simulink model "TetheredHelicopterControlAlgorithm"  (R2019a)
settings: Solver=ode5  StartTime=0.0  StopTime=50  FixedStep=0.01  RelTol=1e-3  AbsTol=1e-6
values from neighbouring files (symbols this model uses):
  Al = A    [Luenberg_matrix_calc.m]
  Bl = B    [Luenberg_matrix_calc.m]
  Cl = [1 0 0; 0 0 1]    [Luenberg_matrix_calc.m]
  fGain = KK(1)    [lqr_pitch.m]
  fi_0 = -0.63    [exp_pitch.m]    (also in linearization.m)
  L = transpose(place(transpose(Al),transpose(Cl),[-100.01,-100.02,-100.03]))    [Luenberg_matrix_calc.m]
  nGain = KK(3)    [lqr_pitch.m]
  pn1 = 1181    [lqr_eq_points.m]
  pn2 = -1053    [lqr_eq_points.m]
  pn3 = 990.5    [lqr_eq_points.m]
  pn4 = 1860    [lqr_eq_points.m]
  pu1 = 0.1721    [lqr_eq_points.m]
  pu2 = -0.1742    [lqr_eq_points.m]
  pu3 = 0.3003    [lqr_eq_points.m]
  pu4 = 0.364    [lqr_eq_points.m]
  wGain = KK(2)    [lqr_pitch.m]
undefined symbols (not defined in the file or in its folder): RTDAC4PCIBaseAddress
libraries: simulink x1, powerlib_meascontrol x1
settings Model: SimulationMode=external  ExtModeTrigDuration=12000  ExtModeTrigLevel=0.400000  Creator=jims  LastModifiedBy=User
settings SolverCC: AutoScaleAbsTol=off
settings DataIOCC: ExternalInput=[]  InitialState=[]  MaxDataPoints=5000  SaveFormat=Array  SignalLoggingSaveFormat=ModelDataLogs  SaveOutput=off  SaveTime=off  ReturnWorkspaceOutputs=off  SignalLoggingName=sigsOut
settings OptimizationCC: BooleanDataType=off  ExpressionDepthLimit=2147483647  InitFltsAndDblsToZero=on  LifeSpan=inf
settings DebuggingCC: SaveWithParameterizedLinksMsg=none  UnderspecifiedInitializationDetection=Classic  MergeDetectMultiDrivingBlocksExec=none  SignalResolutionControl=TryResolveAllWithWarning  MultiTaskDSMMsg=warning  MultiTaskCondExecSysMsg=none  IntegerOverflowMsg=none  FcnCallInpInsideContextMsg=warning  StateNameClashWarn=warning  SFUnexpectedBacktrackingDiag=warning  SFNoUnconditionalDefaultTransitionDiag=warning  SFExecutionAtInitializationDiag=none  IntegerSaturationMsg=none  ArithmeticOperatorsInVariantConditions=warning
settings HardwareCC: ProdBitPerLong=64  ProdLargestAtomicFloat=None  ProdHWDeviceType=Intel->x86-64  TargetBitPerLong=64  TargetBitPerPointer=64  TargetIntDivRoundTo=Zero  TargetEndianess=LittleEndian  TargetWordSize=64  TargetHWDeviceType=Intel->x86-64
settings ModelReferenceCC: PropagateSignalLabelsOutOfModel=off
settings SFSimCC: SimUseLocalCustomCode=off
settings RTWCC: SystemTargetFile=rtwin.tlc  TemplateMakefile=rtwin.tmf  Description=Real-Time Windows Target  RTWUseLocalCustomCode=off
settings CodeAppCC: StateflowObjectComments=on
settings TargetCC: TargetFcnLib=ansi_tfl_tmw.mat  TargetPreCompLibLocation=C:\Program Files\MATLAB\R2015aSP1\toolbox\sldrt\lib\win64  ModelReferenceCompliant=off  CompOptLevelCompliant=off  PreserveStateflowLocalDataDimensions=off
settings ConfigComp: CovMetricSettings=dw  CovHtmlReporting=on  CovSaveCumulativeToWorkspaceVar=on  CovSaveSingleToWorkspaceVar=on  CovExternalEMLEnable=off  CovSFcnEnable=off

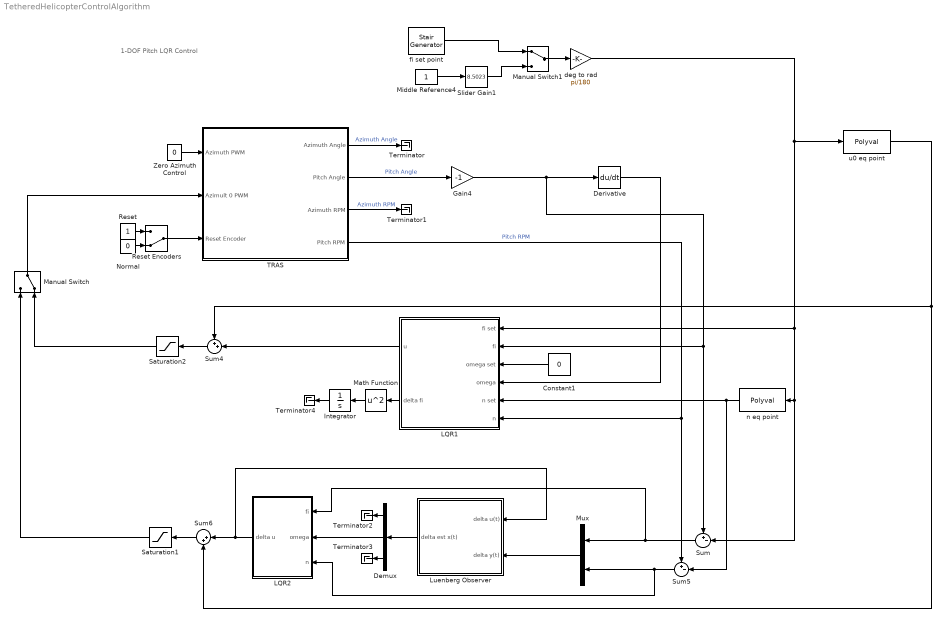
== system TetheredHelicopterControlAlgorithm ==
  note: 1-DOF Pitch LQR Control
  Constant1 : Constant  Value=0
  Demux : Demux  Outputs=3
  Derivative : Derivative
  Gain4 : Gain  Gain=-1
  Integrator : Integrator
  LQR1 : Subsystem
  "LQR2 " : Subsystem
  Luenberg Observer : Subsystem
  Manual Switch : ManualSwitch  CurrentSetting=0
  Manual Switch1 : ManualSwitch
  Math Function : Math  Operator=square  SaturateOnIntegerOverflow=on
  Middle Reference4 : Constant
  Mux : Mux  Inputs=2
  Normal : Constant  Value=0
  Reset : Constant
  Reset Encoders : ManualSwitch  CurrentSetting=0
  Saturation1 : Saturate  UpperLimit=1  LowerLimit=-1
  Saturation2 : Saturate  UpperLimit=1  LowerLimit=-1
  Slider Gain1 : simulink/Math Operations/Slider Gain  gain=8.5023  low=-45  high=45
  Sum : Sum  Inputs=+-|
  Sum4 : Sum  Inputs=++|  SaturateOnIntegerOverflow=on  InputSameDT=on  OutDataTypeStr=Inherit: Same as first input
  Sum5 : Sum  Inputs=+-|
  Sum6 : Sum  Inputs=|++  SaturateOnIntegerOverflow=on  InputSameDT=on  OutDataTypeStr=Inherit: Same as first input
  TRAS : Subsystem  mask{BaseAddress=RTDAC4PCIBaseAddress, T0=0.01}
      mask prompts: BaseAddress "Base Address:"; T0 "Sampling Period:"
      mask Display: image(imread('TRAS.JPG'))
  Terminator{,1..4} (5 alike) : Terminator
  Zero Azimuth Control : Constant  Value=0
  deg to rad : Gain  Gain=pi/180
  fi set point : powerlib_meascontrol/Pulse & Signal Generators/Stair Generator  t=[0 10 20 28 34 42]  e=[0 10 -20 20 -10 30]  Ts=0
      settings: SourceProductName=Simscape Electrical
  n eq point : Polyval  Coefs=[pn1 pn2 pn3 pn4]
  u0 eq point : Polyval  Coefs=[pu1 pu2 pu3 pu4]
  wires:
  TRAS/1(Azimuth Angle) -> Terminator/1  "Azimuth Angle"
  TRAS/2(Pitch Angle) -> Gain4/1  "Pitch Angle"
  TRAS/3(Azimuth RPM) -> Terminator1/1  "Azimuth RPM"
  Normal/1 -> Reset Encoders/2
  Reset/1 -> Reset Encoders/1
  Reset Encoders/1 -> TRAS/3(Reset Encoder)
  Zero Azimuth Control/1 -> TRAS/1(Azimuth PWM)
  TRAS/4(Pitch RPM) -> Sum5/1, LQR1/6(n)  "Pitch RPM"
  Gain4/1 -> Derivative/1, Sum/1, LQR1/2(fi)
  Constant1/1 -> LQR1/3(omega set)
  n eq point/1 -> LQR1/5(n set), Sum5/2
  Sum4/1 -> Saturation2/1
  Manual Switch1/1 -> deg to rad/1
  LQR1/1(u) -> Sum4/2
  Derivative/1 -> LQR1/4(omega)
  LQR1/2(delta fi) -> Math Function/1
  Math Function/1 -> Integrator/1
  Integrator/1 -> Terminator4/1
  u0 eq point/1 -> Sum4/1, Sum6/2
  Sum5/1 -> "LQR2 "/3(n), Mux/2
  Mux/1 -> Luenberg Observer/2(delta y(t))
  Luenberg Observer/1(delta est x(t)) -> Demux/1
  Sum6/1 -> Saturation1/1
  Saturation1/1 -> Manual Switch/1
  "LQR2 "/1("delta u ") -> Luenberg Observer/1(delta u(t)), Sum6/1
  Manual Switch/1 -> TRAS/2(Azimult 0 PWM)
  Saturation2/1 -> Manual Switch/2
  Middle Reference4/1 -> Slider Gain1/1
  Slider Gain1/1 -> Manual Switch1/2
  fi set point/1 -> Manual Switch1/1
  deg to rad/1 -> Sum/2, n eq point/1, LQR1/1(fi set), u0 eq point/1
  Sum/1 -> Mux/1, "LQR2 "/1(fi)
  Demux/2 -> "LQR2 "/2(omega)
  Demux/1 -> Terminator2/1
  Demux/3 -> Terminator3/1

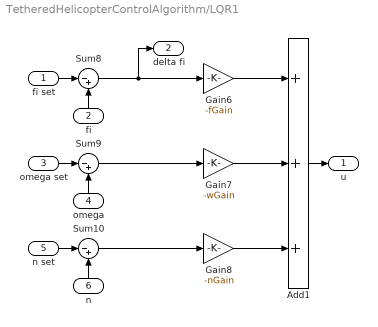
== system TetheredHelicopterControlAlgorithm/LQR1 ==
  fi set : Inport
  fi : Inport  Port=2
  omega set : Inport  Port=3
  omega : Inport  Port=4
  n set : Inport  Port=5
  n : Inport  Port=6
  Add1 : Sum  Inputs=+++
  Gain6 : Gain  Gain=-fGain
  Gain7 : Gain  Gain=-wGain
  Gain8 : Gain  Gain=-nGain
  Sum10 : Sum  Inputs=|-+
  Sum8 : Sum  Inputs=|-+
  Sum9 : Sum  Inputs=|-+
  u : Outport
  delta fi : Outport  Port=2
  wires:
  Gain7/1 -> Add1/2
  Sum8/1 -> delta fi/1, Gain6/1
  Sum9/1 -> Gain7/1
  Gain6/1 -> Add1/1
  Sum10/1 -> Gain8/1
  Gain8/1 -> Add1/3
  fi/1 -> Sum8/2
  n/1 -> Sum10/2
  n set/1 -> Sum10/1
  omega set/1 -> Sum9/1
  omega/1 -> Sum9/2
  Add1/1 -> u/1
  fi set/1 -> Sum8/1

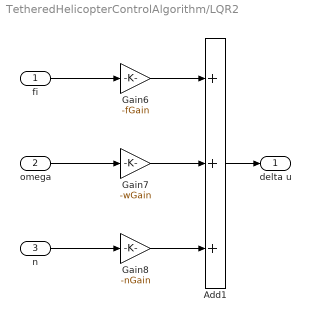
== system TetheredHelicopterControlAlgorithm/LQR2  ==
  fi : Inport
  omega : Inport  Port=2
  n : Inport  Port=3
  Add1 : Sum  Inputs=+++
  Gain6 : Gain  Gain=-fGain
  Gain7 : Gain  Gain=-wGain
  Gain8 : Gain  Gain=-nGain
  "delta u " : Outport
  wires:
  n/1 -> Gain8/1
  Gain7/1 -> Add1/2
  omega/1 -> Gain7/1
  Gain6/1 -> Add1/1
  fi/1 -> Gain6/1
  Add1/1 -> "delta u "/1
  Gain8/1 -> Add1/3

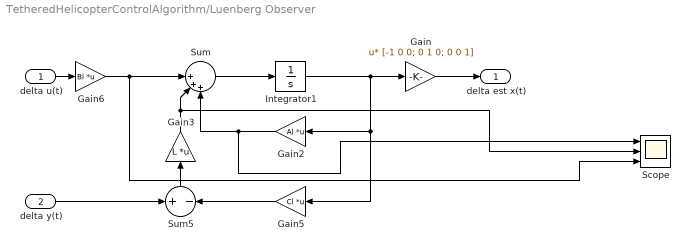
== system TetheredHelicopterControlAlgorithm/Luenberg Observer ==
  delta u(t) : Inport
  delta y(t) : Inport  Port=2
  Gain : Gain  Gain=[-1 0 0; 0 1 0; 0 0 1]  Multiplication=Matrix(u*K)
  Gain2 : Gain  Gain=Al  Multiplication=Matrix(K*u) (u vector)
  Gain3 : Gain  Gain=L  Multiplication=Matrix(K*u) (u vector)
  Gain5 : Gain  Gain=Cl  Multiplication=Matrix(K*u) (u vector)
  Gain6 : Gain  Gain=Bl  Multiplication=Matrix(K*u) (u vector)
  Integrator1 : Integrator  InitialCondition=[fi_0 0 0]  UpperSaturationLimit=auto
  Scope : Scope  NumInputPorts=3
  Sum : Sum  Inputs=||+++
  Sum5 : Sum  Inputs=+|-
  delta est x(t) : Outport
  wires:
  Gain3/1 -> Scope/2, Sum/2
  Gain5/1 -> Sum5/2
  delta y(t)/1 -> Sum5/1
  Gain6/1 -> Scope/3, Sum/1
  Sum5/1 -> Gain3/1
  delta u(t)/1 -> Gain6/1
  Sum/1 -> Integrator1/1
  Gain2/1 -> Scope/1, Sum/3
  Integrator1/1 -> Gain/1, Gain5/1, Gain2/1
  Gain/1 -> delta est x(t)/1

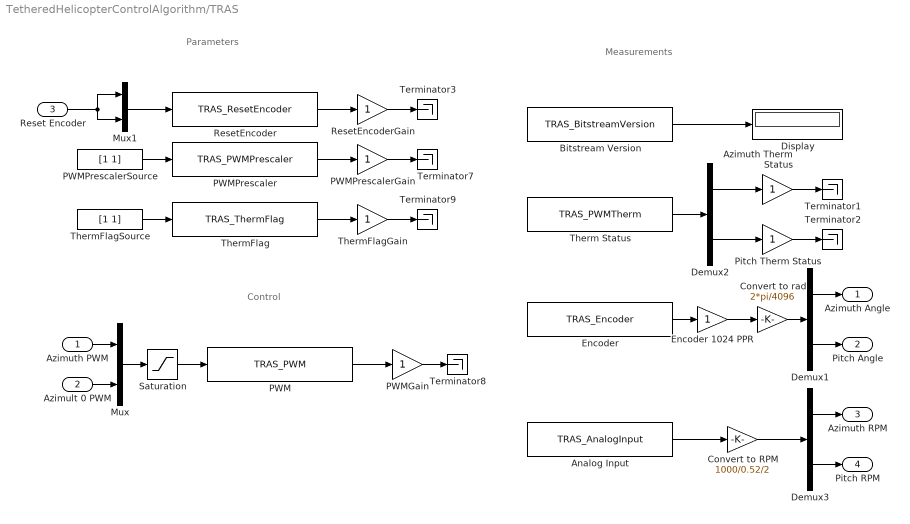
== system TetheredHelicopterControlAlgorithm/TRAS ==
  note: Parameters
  note: Control
  note: Measurements
  Azimuth PWM : Inport
  Azimult 0 PWM : Inport  Port=2
  Reset Encoder : Inport  Port=3
  Analog Input : S-Function  FunctionName=TRAS_AnalogInput  Parameters=BaseAddress, [0 1], [1 1], T0  SFunctionDeploymentMode=off  EnableBusSupport=off
  Azimuth Therm Status : Gain  SaturateOnIntegerOverflow=on  OutDataTypeStr=Inherit: Same as input  ParamDataTypeStr=Inherit: Same as input
  Bitstream Version : S-Function  FunctionName=TRAS_BitstreamVersion  Parameters=BaseAddress, T0  SFunctionDeploymentMode=off  EnableBusSupport=off
  Convert to RPM : Gain  Gain=1000/0.52/2  SaturateOnIntegerOverflow=on  OutDataTypeStr=Inherit: Same as input  ParamDataTypeStr=Inherit: Same as input
  Convert to rad : Gain  Gain=2*pi/4096  SaturateOnIntegerOverflow=on  OutDataTypeStr=Inherit: Same as input  ParamDataTypeStr=Inherit: Same as input
  Demux1 : Demux  Outputs=2
  Demux2 : Demux  Outputs=2
  Demux3 : Demux  Outputs=2
  Display : Display
  Encoder : S-Function  FunctionName=TRAS_Encoder  Parameters=BaseAddress, T0  SFunctionDeploymentMode=off  EnableBusSupport=off
  Encoder 1024 PPR : Gain  SaturateOnIntegerOverflow=on  OutDataTypeStr=Inherit: Same as input  ParamDataTypeStr=Inherit: Same as input
  Mux : Mux  Inputs=2
  Mux1 : Mux  Inputs=2
  PWM : S-Function  FunctionName=TRAS_PWM  Parameters=BaseAddress, T0  SFunctionDeploymentMode=off  EnableBusSupport=off
  PWMGain : Gain  SaturateOnIntegerOverflow=on  OutDataTypeStr=Inherit: Same as input  ParamDataTypeStr=Inherit: Same as input
  PWMPrescaler : S-Function  FunctionName=TRAS_PWMPrescaler  Parameters=BaseAddress, T0  SFunctionDeploymentMode=off  EnableBusSupport=off
  PWMPrescalerGain : Gain  SaturateOnIntegerOverflow=on  OutDataTypeStr=Inherit: Same as input  ParamDataTypeStr=Inherit: Same as input
  PWMPrescalerSource : Constant  Value=[1 1]
  Pitch Therm Status : Gain  SaturateOnIntegerOverflow=on  OutDataTypeStr=Inherit: Same as input  ParamDataTypeStr=Inherit: Same as input
  ResetEncoder : S-Function  FunctionName=TRAS_ResetEncoder  Parameters=BaseAddress, T0  SFunctionDeploymentMode=off  EnableBusSupport=off
  ResetEncoderGain : Gain  SaturateOnIntegerOverflow=on  OutDataTypeStr=Inherit: Same as input  ParamDataTypeStr=Inherit: Same as input
  Saturation : Saturate  UpperLimit=1  LowerLimit=-1
  Terminator{1..3,7..9} (6 alike) : Terminator
  Therm Status : S-Function  FunctionName=TRAS_PWMTherm  Parameters=BaseAddress, T0  SFunctionDeploymentMode=off  EnableBusSupport=off
  "ThermFlag " : S-Function  FunctionName=TRAS_ThermFlag  Parameters=BaseAddress, T0  SFunctionDeploymentMode=off  EnableBusSupport=off
  ThermFlagGain : Gain  SaturateOnIntegerOverflow=on  OutDataTypeStr=Inherit: Same as input  ParamDataTypeStr=Inherit: Same as input
  ThermFlagSource : Constant  Value=[1 1]
  Azimuth Angle : Outport  InitialOutput=0
  Pitch Angle : Outport  Port=2  InitialOutput=0
  Azimuth RPM : Outport  Port=3  InitialOutput=0
  Pitch RPM : Outport  Port=4  InitialOutput=0
  wires:
  Encoder 1024 PPR/1 -> Convert to rad/1
  Encoder/1 -> Encoder 1024 PPR/1
  Saturation/1 -> PWM/1
  Mux/1 -> Saturation/1
  PWM/1 -> PWMGain/1
  PWMGain/1 -> Terminator8/1
  ResetEncoder/1 -> ResetEncoderGain/1
  PWMPrescaler/1 -> PWMPrescalerGain/1
  Mux1/1 -> ResetEncoder/1
  PWMPrescalerSource/1 -> PWMPrescaler/1
  ResetEncoderGain/1 -> Terminator3/1
  PWMPrescalerGain/1 -> Terminator7/1
  Azimult 0 PWM/1 -> Mux/2
  Azimuth PWM/1 -> Mux/1
  Demux1/2 -> Pitch Angle/1
  Convert to rad/1 -> Demux1/1
  Demux1/1 -> Azimuth Angle/1
  Therm Status/1 -> Demux2/1
  Demux2/2 -> Pitch Therm Status/1
  Demux2/1 -> Azimuth Therm Status/1
  Azimuth Therm Status/1 -> Terminator1/1
  Pitch Therm Status/1 -> Terminator2/1
  Bitstream Version/1 -> Display/1
  Analog Input/1 -> Convert to RPM/1
  Demux3/2 -> Pitch RPM/1
  Demux3/1 -> Azimuth RPM/1
  Reset Encoder/1 -> Mux1/1, Mux1/2
  Convert to RPM/1 -> Demux3/1
  "ThermFlag "/1 -> ThermFlagGain/1
  ThermFlagSource/1 -> "ThermFlag "/1
  ThermFlagGain/1 -> Terminator9/1
